simulink library "halout"  (R2021b)
settings: Solver=VariableStepAuto  StartTime=0.0  StopTime=10.0  RelTol=1e-3
undefined symbols (not defined in the file): C_TASK_5MS_S, FALSE, KHAL_CAN1FD1APS3E2E_flg, KHAL_CAN1FD1APS3TxReq_flg, KHAL_CAN1FD1VCU2E2E_flg, KHAL_CAN1FD1VCU2TxReq_flg, KHAL_CAN1FD1VCU3E2E_flg, KHAL_CAN1FD1VCU3TxReq_flg, KHAL_CAN1TxReq_flg, KHAL_CAN1VMCFCM1E2E_flg, KHAL_CAN1VMCFCM1TxReq_flg, KHAL_CAN2TxReq_flg, KHAL_CAN3FD3VCU1toNIDECTxReq_flg, KHAL_CAN3FD3VCU1TxReq_flg, KHAL_CAN3FD3VCU2E2E_flg, KHAL_CAN3FD3VCU2toNIDECE2E_flg, KHAL_CAN3FD3VCU2toNIDECTxReq_flg, KHAL_CAN3FD3VCU2TxReq_flg, KHAL_CAN3TxReq_flg, KHAL_CAN4FD4CE1000E2E_flg, KHAL_CAN4FD4CE1000TxReq_flg, KHAL_CAN4TxReq_flg, KHAL_CAN5TxReq_flg, KHAL_CAN6FD6APS3E2E_flg, KHAL_CAN6FD6APS3TxReq_flg, KHAL_CAN6FD6VCU2E2E_flg, KHAL_CAN6FD6VCU2TxReq_flg, KHAL_CAN6TxReq_flg, ONE_INT, TRUE, ZERO_INT
libraries: FVT_lib x551, simulink x244
(part 19 of 26)

== system halout/HAL_OUT/CAN3/FD3_BCM1_0x216/Dimmer ==
  Dimmer : Inport
  Data Type Conversion : DataTypeConversion  OutDataTypeStr=uint8  RndMeth=Round
  CAN3_Dimmer : Outport
  wires:
  Data Type Conversion/1 -> CAN3_Dimmer/1
  Dimmer/1 -> Data Type Conversion/1

== system halout/HAL_OUT/CAN3/FD3_BCM1_0x216/DimmerEN ==
  DimmerEN : Inport
  Data Type Conversion : DataTypeConversion  OutDataTypeStr=uint8  RndMeth=Round
  CAN3_DimmerEN : Outport
  wires:
  Data Type Conversion/1 -> CAN3_DimmerEN/1
  DimmerEN/1 -> Data Type Conversion/1

== system halout/HAL_OUT/CAN3/FD3_BCM1_0x216/DoorLockIND ==
  DoorLockIND : Inport
  Data Type Conversion : DataTypeConversion  OutDataTypeStr=uint8  RndMeth=Round
  CAN3_DoorLockIND : Outport
  wires:
  Data Type Conversion/1 -> CAN3_DoorLockIND/1
  DoorLockIND/1 -> Data Type Conversion/1

== system halout/HAL_OUT/CAN3/FD3_BCM1_0x216/DrDoorSW ==
  DrDoorSW : Inport
  Data Type Conversion : DataTypeConversion  OutDataTypeStr=uint8  RndMeth=Round
  CAN3_DrDoorSW : Outport
  wires:
  Data Type Conversion/1 -> CAN3_DrDoorSW/1
  DrDoorSW/1 -> Data Type Conversion/1

== system halout/HAL_OUT/CAN3/FD3_BCM1_0x216/FrChargingDoorCtrl ==
  FrChargingDoorCtrl : Inport
  Data Type Conversion : DataTypeConversion  OutDataTypeStr=uint8  RndMeth=Round
  CAN3_Fr_ChargingDoorCtrl : Outport
  wires:
  Data Type Conversion/1 -> CAN3_Fr_ChargingDoorCtrl/1
  FrChargingDoorCtrl/1 -> Data Type Conversion/1

== system halout/HAL_OUT/CAN3/FD3_BCM1_0x216/FrFogLamp ==
  FrFogLamp : Inport
  Data Type Conversion : DataTypeConversion  OutDataTypeStr=uint8  RndMeth=Round
  CAN3_Fr_FogLamp : Outport
  wires:
  Data Type Conversion/1 -> CAN3_Fr_FogLamp/1
  FrFogLamp/1 -> Data Type Conversion/1

== system halout/HAL_OUT/CAN3/FD3_BCM1_0x216/FrWiperH ==
  FrWiperH : Inport
  Data Type Conversion : DataTypeConversion  OutDataTypeStr=uint8  RndMeth=Round
  CAN3_Fr_Wiper_H : Outport
  wires:
  Data Type Conversion/1 -> CAN3_Fr_Wiper_H/1
  FrWiperH/1 -> Data Type Conversion/1

== system halout/HAL_OUT/CAN3/FD3_BCM1_0x216/FrWiperL ==
  FrWiperL : Inport
  Data Type Conversion : DataTypeConversion  OutDataTypeStr=uint8  RndMeth=Round
  CAN3_Fr_Wiper_L : Outport
  wires:
  Data Type Conversion/1 -> CAN3_Fr_Wiper_L/1
  FrWiperL/1 -> Data Type Conversion/1

== system halout/HAL_OUT/CAN3/FD3_BCM1_0x216/HBeam ==
  HBeam : Inport
  Data Type Conversion : DataTypeConversion  OutDataTypeStr=uint8  RndMeth=Round
  CAN3_H_Beam : Outport
  wires:
  Data Type Conversion/1 -> CAN3_H_Beam/1
  HBeam/1 -> Data Type Conversion/1

== system halout/HAL_OUT/CAN3/FD3_BCM1_0x216/HazardSW ==
  HazardSW : Inport
  Data Type Conversion : DataTypeConversion  OutDataTypeStr=uint8  RndMeth=Round
  CAN3_HazardSW : Outport
  wires:
  Data Type Conversion/1 -> CAN3_HazardSW/1
  HazardSW/1 -> Data Type Conversion/1

== system halout/HAL_OUT/CAN3/FD3_BCM1_0x216/HoodSW ==
  HoodSW : Inport
  Data Type Conversion : DataTypeConversion  OutDataTypeStr=uint8  RndMeth=Round
  CAN3_HoodSW : Outport
  wires:
  Data Type Conversion/1 -> CAN3_HoodSW/1
  HoodSW/1 -> Data Type Conversion/1

== system halout/HAL_OUT/CAN3/FD3_BCM1_0x216/HornCtrl ==
  HornCtrl : Inport
  Data Type Conversion : DataTypeConversion  OutDataTypeStr=uint8  RndMeth=Round
  CAN3_HornCtrl : Outport
  wires:
  Data Type Conversion/1 -> CAN3_HornCtrl/1
  HornCtrl/1 -> Data Type Conversion/1

== system halout/HAL_OUT/CAN3/FD3_BCM1_0x216/LAPMWdwEnable ==
  LAPMWdwEnable : Inport
  Data Type Conversion : DataTypeConversion  OutDataTypeStr=uint8  RndMeth=Round
  CAN3_L_APM_WdwEnable : Outport
  wires:
  Data Type Conversion/1 -> CAN3_L_APM_WdwEnable/1
  LAPMWdwEnable/1 -> Data Type Conversion/1

== system halout/HAL_OUT/CAN3/FD3_BCM1_0x216/LBSD ==
  LBSD : Inport
  Data Type Conversion : DataTypeConversion  OutDataTypeStr=uint8  RndMeth=Round
  CAN3_LBSD : Outport
  wires:
  Data Type Conversion/1 -> CAN3_LBSD/1
  LBSD/1 -> Data Type Conversion/1

== system halout/HAL_OUT/CAN3/FD3_BCM1_0x216/LBeam ==
  LBeam : Inport
  Data Type Conversion : DataTypeConversion  OutDataTypeStr=uint8  RndMeth=Round
  CAN3_L_Beam : Outport
  wires:
  Data Type Conversion/1 -> CAN3_L_Beam/1
  LBeam/1 -> Data Type Conversion/1

== system halout/HAL_OUT/CAN3/FD3_BCM1_0x216/LDRL ==
  LDRL : Inport
  Data Type Conversion : DataTypeConversion  OutDataTypeStr=uint8  RndMeth=Round
  CAN3_LDRL : Outport
  wires:
  Data Type Conversion/1 -> CAN3_LDRL/1
  LDRL/1 -> Data Type Conversion/1

== system halout/HAL_OUT/CAN3/FD3_BCM1_0x216/LTurnLP ==
  LTurnLP : Inport
  Data Type Conversion : DataTypeConversion  OutDataTypeStr=uint8  RndMeth=Round
  CAN3_LTurnLP : Outport
  wires:
  Data Type Conversion/1 -> CAN3_LTurnLP/1
  LTurnLP/1 -> Data Type Conversion/1

== system halout/HAL_OUT/CAN3/FD3_BCM1_0x216/LockSetting ==
  LockSetting : Inport
  Data Type Conversion : DataTypeConversion  OutDataTypeStr=uint8  RndMeth=Round
  CAN3_LockSetting : Outport
  wires:
  Data Type Conversion/1 -> CAN3_LockSetting/1
  LockSetting/1 -> Data Type Conversion/1

== system halout/HAL_OUT/CAN3/FD3_BCM1_0x216/MirrorCtrl ==
  MirrorCtrl : Inport
  Data Type Conversion : DataTypeConversion  OutDataTypeStr=uint8  RndMeth=Round
  CAN3_MirrorCtrl : Outport
  wires:
  Data Type Conversion/1 -> CAN3_MirrorCtrl/1
  MirrorCtrl/1 -> Data Type Conversion/1

== system halout/HAL_OUT/CAN3/FD3_BCM1_0x216/MirrorDefog ==
  MirrorDefog : Inport
  Data Type Conversion : DataTypeConversion  OutDataTypeStr=uint8  RndMeth=Round
  CAN3_MirrorDefog : Outport
  wires:
  Data Type Conversion/1 -> CAN3_MirrorDefog/1
  MirrorDefog/1 -> Data Type Conversion/1

== system halout/HAL_OUT/CAN3/FD3_BCM1_0x216/PosLamp ==
  PosLamp : Inport
  Data Type Conversion : DataTypeConversion  OutDataTypeStr=uint8  RndMeth=Round
  CAN3_PosLamp : Outport
  wires:
  Data Type Conversion/1 -> CAN3_PosLamp/1
  PosLamp/1 -> Data Type Conversion/1

== system halout/HAL_OUT/CAN3/FD3_BCM1_0x216/PsDoorSW ==
  PsDoorSW : Inport
  Data Type Conversion : DataTypeConversion  OutDataTypeStr=uint8  RndMeth=Round
  CAN3_PsDoorSW : Outport
  wires:
  Data Type Conversion/1 -> CAN3_PsDoorSW/1
  PsDoorSW/1 -> Data Type Conversion/1

== system halout/HAL_OUT/CAN3/FD3_BCM1_0x216/RBSD ==
  RBSD : Inport
  Data Type Conversion : DataTypeConversion  OutDataTypeStr=uint8  RndMeth=Round
  CAN3_RBSD : Outport
  wires:
  Data Type Conversion/1 -> CAN3_RBSD/1
  RBSD/1 -> Data Type Conversion/1

== system halout/HAL_OUT/CAN3/FD3_BCM1_0x216/RDRL ==
  RDRL : Inport
  Data Type Conversion : DataTypeConversion  OutDataTypeStr=uint8  RndMeth=Round
  CAN3_RDRL : Outport
  wires:
  Data Type Conversion/1 -> CAN3_RDRL/1
  RDRL/1 -> Data Type Conversion/1

== system halout/HAL_OUT/CAN3/FD3_BCM1_0x216/RLDoorSW ==
  RLDoorSW : Inport
  Data Type Conversion : DataTypeConversion  OutDataTypeStr=uint8  RndMeth=Round
  CAN3_RLDoorSW : Outport
  wires:
  Data Type Conversion/1 -> CAN3_RLDoorSW/1
  RLDoorSW/1 -> Data Type Conversion/1

== system halout/HAL_OUT/CAN3/FD3_BCM1_0x216/RRDoorSW ==
  RRDoorSW : Inport
  Data Type Conversion : DataTypeConversion  OutDataTypeStr=uint8  RndMeth=Round
  CAN3_RRDoorSW : Outport
  wires:
  Data Type Conversion/1 -> CAN3_RRDoorSW/1
  RRDoorSW/1 -> Data Type Conversion/1

== system halout/HAL_OUT/CAN3/FD3_BCM1_0x216/RTurnLP ==
  RTurnLP : Inport
  Data Type Conversion : DataTypeConversion  OutDataTypeStr=uint8  RndMeth=Round
  CAN3_RTurnLP : Outport
  wires:
  Data Type Conversion/1 -> CAN3_RTurnLP/1
  RTurnLP/1 -> Data Type Conversion/1

== system halout/HAL_OUT/CAN3/FD3_BCM1_0x216/ReverseLamp ==
  ReverseLamp : Inport
  Data Type Conversion : DataTypeConversion  OutDataTypeStr=uint8  RndMeth=Round
  CAN3_ReverseLamp : Outport
  wires:
  Data Type Conversion/1 -> CAN3_ReverseLamp/1
  ReverseLamp/1 -> Data Type Conversion/1

== system halout/HAL_OUT/CAN3/FD3_BCM1_0x216/RoomLampH ==
  RoomLampH : Inport
  Data Type Conversion : DataTypeConversion  OutDataTypeStr=uint8  RndMeth=Round
  CAN3_RoomLampH : Outport
  wires:
  Data Type Conversion/1 -> CAN3_RoomLampH/1
  RoomLampH/1 -> Data Type Conversion/1

== system halout/HAL_OUT/CAN3/FD3_BCM1_0x216/RoomLampL ==
  RoomLampL : Inport
  Data Type Conversion : DataTypeConversion  OutDataTypeStr=uint8  RndMeth=Round
  CAN3_RoomLampL : Outport
  wires:
  Data Type Conversion/1 -> CAN3_RoomLampL/1
  RoomLampL/1 -> Data Type Conversion/1

== system halout/HAL_OUT/CAN3/FD3_BCM1_0x216/RrChargingDoorCtrl ==
  RrChargingDoorCtrl : Inport
  Data Type Conversion : DataTypeConversion  OutDataTypeStr=uint8  RndMeth=Round
  CAN3_Rr_ChargingDoorCtrl : Outport
  wires:
  Data Type Conversion/1 -> CAN3_Rr_ChargingDoorCtrl/1
  RrChargingDoorCtrl/1 -> Data Type Conversion/1

== system halout/HAL_OUT/CAN3/FD3_BCM1_0x216/RrDefog ==
  RrDefog : Inport
  Data Type Conversion : DataTypeConversion  OutDataTypeStr=uint8  RndMeth=Round
  CAN3_Rr_Defog : Outport
  wires:
  Data Type Conversion/1 -> CAN3_Rr_Defog/1
  RrDefog/1 -> Data Type Conversion/1

== system halout/HAL_OUT/CAN3/FD3_BCM1_0x216/RrFogLamp ==
  RrFogLamp : Inport
  Data Type Conversion : DataTypeConversion  OutDataTypeStr=uint8  RndMeth=Round
  CAN3_Rr_FogLamp : Outport
  wires:
  Data Type Conversion/1 -> CAN3_Rr_FogLamp/1
  RrFogLamp/1 -> Data Type Conversion/1

== system halout/HAL_OUT/CAN3/FD3_BCM1_0x216/RrWiper ==
  RrWiper : Inport
  Data Type Conversion : DataTypeConversion  OutDataTypeStr=uint8  RndMeth=Round
  CAN3_Rr_Wiper : Outport
  wires:
  Data Type Conversion/1 -> CAN3_Rr_Wiper/1
  RrWiper/1 -> Data Type Conversion/1

== system halout/HAL_OUT/CAN3/FD3_BCM1_0x216/TailgateHDSW ==
  TailgateHDSW : Inport
  Data Type Conversion : DataTypeConversion  OutDataTypeStr=uint8  RndMeth=Round
  CAN3_TailgateHDSW : Outport
  wires:
  Data Type Conversion/1 -> CAN3_TailgateHDSW/1
  TailgateHDSW/1 -> Data Type Conversion/1

== system halout/HAL_OUT/CAN3/FD3_BCM1_0x216/TailgateRemote ==
  TailgateRemote : Inport
  Data Type Conversion : DataTypeConversion  OutDataTypeStr=uint8  RndMeth=Round
  CAN3_TailgateRemote : Outport
  wires:
  Data Type Conversion/1 -> CAN3_TailgateRemote/1
  TailgateRemote/1 -> Data Type Conversion/1

== system halout/HAL_OUT/CAN3/FD3_BCM1_0x216/TailgateSW ==
  TailgateSW : Inport
  Data Type Conversion : DataTypeConversion  OutDataTypeStr=uint8  RndMeth=Round
  CAN3_Tailgate_SW : Outport
  wires:
  Data Type Conversion/1 -> CAN3_Tailgate_SW/1
  TailgateSW/1 -> Data Type Conversion/1

== system halout/HAL_OUT/CAN3/FD3_BCM1_0x216/TrunkRel ==
  TrunkRel : Inport
  Data Type Conversion : DataTypeConversion  OutDataTypeStr=uint8  RndMeth=Round
  CAN3_TrunkRel : Outport
  wires:
  Data Type Conversion/1 -> CAN3_TrunkRel/1
  TrunkRel/1 -> Data Type Conversion/1

== system halout/HAL_OUT/CAN3/FD3_BCM1_0x216/WasherCtrl ==
  WasherCtrl : Inport
  Data Type Conversion : DataTypeConversion  OutDataTypeStr=uint8  RndMeth=Round
  CAN3_WasherCtrl : Outport
  wires:
  Data Type Conversion/1 -> CAN3_WasherCtrl/1
  WasherCtrl/1 -> Data Type Conversion/1

== system halout/HAL_OUT/CAN3/FD3_BCM1_0x216/WiperFixMode ==
  WiperFixMode : Inport
  Data Type Conversion : DataTypeConversion  OutDataTypeStr=uint8  RndMeth=Round
  CAN3_WiperFixMode : Outport
  wires:
  Data Type Conversion/1 -> CAN3_WiperFixMode/1
  WiperFixMode/1 -> Data Type Conversion/1

== system halout/HAL_OUT/CAN3/FD3_C100_0_0x182/BatteryMode ==
  BatteryMode : Inport
  Data Type Conversion : DataTypeConversion  OutDataTypeStr=uint8  RndMeth=Round
  CAN3_BatteryMode : Outport
  wires:
  Data Type Conversion/1 -> CAN3_BatteryMode/1
  BatteryMode/1 -> Data Type Conversion/1

== system halout/HAL_OUT/CAN3/FD3_C100_0_0x182/FrCoolantflow ==
  FrCoolantflow : Inport
  Data Type Conversion : DataTypeConversion  OutDataTypeStr=uint8  RndMeth=Round
  convert_out : FVT_lib/hal/convert_out  gain=0.25  offset=0
  CAN3_Fr_Coolantflow : Outport
  wires:
  Data Type Conversion/1 -> CAN3_Fr_Coolantflow/1
  convert_out/1 -> Data Type Conversion/1
  FrCoolantflow/1 -> convert_out/1

== system halout/HAL_OUT/CAN3/FD3_C100_0_0x182/FrCoolanttemp ==
  FrCoolanttemp : Inport
  Data Type Conversion : DataTypeConversion  OutDataTypeStr=uint16  RndMeth=Round
  convert_out : FVT_lib/hal/convert_out  gain=1  offset=-40
  CAN3_Fr_Coolanttemp : Outport
  wires:
  Data Type Conversion/1 -> CAN3_Fr_Coolanttemp/1
  convert_out/1 -> Data Type Conversion/1
  FrCoolanttemp/1 -> convert_out/1

== system halout/HAL_OUT/CAN3/FD3_C100_0_0x182/RrCoolantflow ==
  RrCoolantflow : Inport
  Data Type Conversion : DataTypeConversion  OutDataTypeStr=uint8  RndMeth=Round
  convert_out : FVT_lib/hal/convert_out  gain=0.25  offset=0
  CAN3_Rr_Coolantflow : Outport
  wires:
  Data Type Conversion/1 -> CAN3_Rr_Coolantflow/1
  convert_out/1 -> Data Type Conversion/1
  RrCoolantflow/1 -> convert_out/1

== system halout/HAL_OUT/CAN3/FD3_C100_0_0x182/RrCoolanttemp ==
  RrCoolanttemp : Inport
  Data Type Conversion : DataTypeConversion  OutDataTypeStr=uint16  RndMeth=Round
  convert_out : FVT_lib/hal/convert_out  gain=1  offset=-40
  CAN3_Rr_Coolanttemp : Outport
  wires:
  Data Type Conversion/1 -> CAN3_Rr_Coolanttemp/1
  convert_out/1 -> Data Type Conversion/1
  RrCoolanttemp/1 -> convert_out/1

== system halout/HAL_OUT/CAN3/FD3_C100_0_0x182/sigCbnPTCPwrAct ==
  sigCbnPTCPwrAct : Inport
  Data Type Conversion : DataTypeConversion  OutDataTypeStr=uint8  RndMeth=Round
  convert_out : FVT_lib/hal/convert_out  gain=50  offset=0
  CAN3_sigCbnPTCPwrAct : Outport
  wires:
  Data Type Conversion/1 -> CAN3_sigCbnPTCPwrAct/1
  convert_out/1 -> Data Type Conversion/1
  sigCbnPTCPwrAct/1 -> convert_out/1

== system halout/HAL_OUT/CAN3/FD3_V2L1_0x374/FDCV2LOBCExtrV2LCmd ==
  FDCV2LOBCExtrV2LCmd : Inport
  Data Type Conversion : DataTypeConversion  OutDataTypeStr=uint8  RndMeth=Round
  CAN3_FDC_V2L_OBCExtrV2L_Cmd : Outport
  wires:
  Data Type Conversion/1 -> CAN3_FDC_V2L_OBCExtrV2L_Cmd/1
  FDCV2LOBCExtrV2LCmd/1 -> Data Type Conversion/1

== system halout/HAL_OUT/CAN3/FD3_V2L1_0x374/FDCV2LOBCIntrV2LCmd ==
  FDCV2LOBCIntrV2LCmd : Inport
  Data Type Conversion : DataTypeConversion  OutDataTypeStr=uint8  RndMeth=Round
  CAN3_FDC_V2L_OBCIntrV2L_Cmd : Outport
  wires:
  Data Type Conversion/1 -> CAN3_FDC_V2L_OBCIntrV2L_Cmd/1
  FDCV2LOBCIntrV2LCmd/1 -> Data Type Conversion/1

== system halout/HAL_OUT/CAN3/FD3_V2L1_0x374/ReqOBCV2LEna ==
  ReqOBCV2LEna : Inport
  Data Type Conversion : DataTypeConversion  OutDataTypeStr=uint8  RndMeth=Round
  CAN3_Req_OBCV2LEna : Outport
  wires:
  Data Type Conversion/1 -> CAN3_Req_OBCV2LEna/1
  ReqOBCV2LEna/1 -> Data Type Conversion/1

== system halout/HAL_OUT/CAN3/FD3_V2L1_0x374/ReqV2LIVIPopup ==
  ReqV2LIVIPopup : Inport
  Data Type Conversion : DataTypeConversion  OutDataTypeStr=uint8  RndMeth=Round
  CAN3_Req_V2L_IVI_Popup : Outport
  wires:
  Data Type Conversion/1 -> CAN3_Req_V2L_IVI_Popup/1
  ReqV2LIVIPopup/1 -> Data Type Conversion/1

== system halout/HAL_OUT/CAN3/FD3_V2L1_0x374/ReqV2LSwOn ==
  ReqV2LSwOn : Inport
  Data Type Conversion : DataTypeConversion  OutDataTypeStr=uint8  RndMeth=Round
  CAN3_Req_V2LSwOn : Outport
  wires:
  Data Type Conversion/1 -> CAN3_Req_V2LSwOn/1
  ReqV2LSwOn/1 -> Data Type Conversion/1

== system halout/HAL_OUT/CAN3/FD3_VCU0_0x1F0/EVCCAplusPwrUpReq ==
  EVCCAplusPwrUpReq : Inport
  Data Type Conversion : DataTypeConversion  OutDataTypeStr=uint8  RndMeth=Round
  CAN3_EVCCAplusPwrUpReq : Outport
  wires:
  Data Type Conversion/1 -> CAN3_EVCCAplusPwrUpReq/1
  EVCCAplusPwrUpReq/1 -> Data Type Conversion/1

== system halout/HAL_OUT/CAN3/FD3_VCU0_0x1F0/FDADC12VDet ==
  FDADC12VDet : Inport
  Data Type Conversion : DataTypeConversion  OutDataTypeStr=uint8  RndMeth=Round
  convert_out : FVT_lib/hal/convert_out  gain=0.1  offset=0
  CAN3_FDADC12VDet : Outport
  wires:
  Data Type Conversion/1 -> CAN3_FDADC12VDet/1
  convert_out/1 -> Data Type Conversion/1
  FDADC12VDet/1 -> convert_out/1

== system halout/HAL_OUT/CAN3/FD3_VCU0_0x1F0/FDADC12VDetAvg ==
  FDADC12VDetAvg : Inport
  Data Type Conversion : DataTypeConversion  OutDataTypeStr=uint8  RndMeth=Round
  convert_out : FVT_lib/hal/convert_out  gain=0.1  offset=0
  CAN3_FDADC12VDetAvg : Outport
  wires:
  Data Type Conversion/1 -> CAN3_FDADC12VDetAvg/1
  convert_out/1 -> Data Type Conversion/1
  FDADC12VDetAvg/1 -> convert_out/1

== system halout/HAL_OUT/CAN3/FD3_VCU0_0x1F0/FDCSYSPmicBootPath ==
  FDCSYSPmicBootPath : Inport
  Data Type Conversion : DataTypeConversion  OutDataTypeStr=uint32  RndMeth=Round
  CAN3_FDC_SYS_PmicBootPath : Outport
  wires:
  Data Type Conversion/1 -> CAN3_FDC_SYS_PmicBootPath/1
  FDCSYSPmicBootPath/1 -> Data Type Conversion/1

== system halout/HAL_OUT/CAN3/FD3_VCU0_0x1F0/FDCVCUActMaxSlideRateSta ==
  FDCVCUActMaxSlideRateSta : Inport
  Data Type Conversion : DataTypeConversion  OutDataTypeStr=uint16  RndMeth=Round
  convert_out : FVT_lib/hal/convert_out  gain=0.01  offset=-150
  CAN3_FDC_VCU_ActMaxSlideRate_Sta : Outport
  wires:
  Data Type Conversion/1 -> CAN3_FDC_VCU_ActMaxSlideRate_Sta/1
  convert_out/1 -> Data Type Conversion/1
  FDCVCUActMaxSlideRateSta/1 -> convert_out/1

== system halout/HAL_OUT/CAN3/FD3_VCU0_0x1F0/FDCVCUAllowMovThdOTASta ==
  FDCVCUAllowMovThdOTASta : Inport
  Data Type Conversion : DataTypeConversion  OutDataTypeStr=uint8  RndMeth=Round
  CAN3_FDC_VCU_AllowMovThd_OTA_Sta : Outport
  wires:
  Data Type Conversion/1 -> CAN3_FDC_VCU_AllowMovThd_OTA_Sta/1
  FDCVCUAllowMovThdOTASta/1 -> Data Type Conversion/1

== system halout/HAL_OUT/CAN3/FD3_VCU0_0x1F0/FDCVCUBOSEnableSta ==
  FDCVCUBOSEnableSta : Inport
  Data Type Conversion : DataTypeConversion  OutDataTypeStr=uint8  RndMeth=Round
  CAN3_FDC_VCU_BOSEnable_Sta : Outport
  wires:
  Data Type Conversion/1 -> CAN3_FDC_VCU_BOSEnable_Sta/1
  FDCVCUBOSEnableSta/1 -> Data Type Conversion/1

== system halout/HAL_OUT/CAN3/FD3_VCU0_0x1F0/FDCVCUBrakeSigMatrixSta ==
  FDCVCUBrakeSigMatrixSta : Inport
  Data Type Conversion : DataTypeConversion  OutDataTypeStr=uint8  RndMeth=Round
  CAN3_FDC_VCU_BrakeSigMatrix_Sta : Outport
  wires:
  Data Type Conversion/1 -> CAN3_FDC_VCU_BrakeSigMatrix_Sta/1
  FDCVCUBrakeSigMatrixSta/1 -> Data Type Conversion/1

== system halout/HAL_OUT/CAN3/FD3_VCU0_0x1F0/FDCVCUBrkPedalPosStaSta ==
  FDCVCUBrkPedalPosStaSta : Inport
  Data Type Conversion : DataTypeConversion  OutDataTypeStr=uint8  RndMeth=Round
  CAN3_FDC_VCU_BrkPedalPosSta_Sta : Outport
  wires:
  Data Type Conversion/1 -> CAN3_FDC_VCU_BrkPedalPosSta_Sta/1
  FDCVCUBrkPedalPosStaSta/1 -> Data Type Conversion/1

== system halout/HAL_OUT/CAN3/FD3_VCU0_0x1F0/FDCVCUCANBrkSW2StaSta ==
  FDCVCUCANBrkSW2StaSta : Inport
  Data Type Conversion : DataTypeConversion  OutDataTypeStr=uint8  RndMeth=Round
  CAN3_FDC_VCU_CANBrkSW2Sta_Sta : Outport
  wires:
  Data Type Conversion/1 -> CAN3_FDC_VCU_CANBrkSW2Sta_Sta/1
  FDCVCUCANBrkSW2StaSta/1 -> Data Type Conversion/1

== system halout/HAL_OUT/CAN3/FD3_VCU0_0x1F0/FDCVCUDTCCarouselSta ==
  FDCVCUDTCCarouselSta : Inport
  Data Type Conversion : DataTypeConversion  OutDataTypeStr=uint8  RndMeth=Round
  CAN3_FDC_VCU_DTCCarousel_Sta : Outport
  wires:
  Data Type Conversion/1 -> CAN3_FDC_VCU_DTCCarousel_Sta/1
  FDCVCUDTCCarouselSta/1 -> Data Type Conversion/1

== system halout/HAL_OUT/CAN3/FD3_VCU0_0x1F0/FDCVCUEAPS1MinSta ==
  FDCVCUEAPS1MinSta : Inport
  Data Type Conversion : DataTypeConversion  OutDataTypeStr=uint8  RndMeth=Round
  convert_out : FVT_lib/hal/convert_out  gain=0.4  offset=0
  CAN3_FDC_VCU_EAPS1Min_Sta : Outport
  wires:
  Data Type Conversion/1 -> CAN3_FDC_VCU_EAPS1Min_Sta/1
  convert_out/1 -> Data Type Conversion/1
  FDCVCUEAPS1MinSta/1 -> convert_out/1

== system halout/HAL_OUT/CAN3/FD3_VCU0_0x1F0/FDCVCUEAPS1RawSta ==
  FDCVCUEAPS1RawSta : Inport
  Data Type Conversion : DataTypeConversion  OutDataTypeStr=uint8  RndMeth=Round
  convert_out : FVT_lib/hal/convert_out  gain=0.4  offset=0
  CAN3_FDC_VCU_EAPS1Raw_Sta : Outport
  wires:
  Data Type Conversion/1 -> CAN3_FDC_VCU_EAPS1Raw_Sta/1
  convert_out/1 -> Data Type Conversion/1
  FDCVCUEAPS1RawSta/1 -> convert_out/1

== system halout/HAL_OUT/CAN3/FD3_VCU0_0x1F0/FDCVCUEAPS2MinSta ==
  FDCVCUEAPS2MinSta : Inport
  Data Type Conversion : DataTypeConversion  OutDataTypeStr=uint8  RndMeth=Round
  convert_out : FVT_lib/hal/convert_out  gain=0.4  offset=0
  CAN3_FDC_VCU_EAPS2Min_Sta : Outport
  wires:
  Data Type Conversion/1 -> CAN3_FDC_VCU_EAPS2Min_Sta/1
  convert_out/1 -> Data Type Conversion/1
  FDCVCUEAPS2MinSta/1 -> convert_out/1

== system halout/HAL_OUT/CAN3/FD3_VCU0_0x1F0/FDCVCUEAPS2RawSta ==
  FDCVCUEAPS2RawSta : Inport
  Data Type Conversion : DataTypeConversion  OutDataTypeStr=uint8  RndMeth=Round
  convert_out : FVT_lib/hal/convert_out  gain=0.4  offset=0
  CAN3_FDC_VCU_EAPS2Raw_Sta : Outport
  wires:
  Data Type Conversion/1 -> CAN3_FDC_VCU_EAPS2Raw_Sta/1
  convert_out/1 -> Data Type Conversion/1
  FDCVCUEAPS2RawSta/1 -> convert_out/1

== system halout/HAL_OUT/CAN3/FD3_VCU0_0x1F0/FDCVCUForcePCmd ==
  FDCVCUForcePCmd : Inport
  Data Type Conversion : DataTypeConversion  OutDataTypeStr=uint8  RndMeth=Round
  CAN3_FDC_VCU_ForceP_Cmd : Outport
  wires:
  Data Type Conversion/1 -> CAN3_FDC_VCU_ForceP_Cmd/1
  FDCVCUForcePCmd/1 -> Data Type Conversion/1

== system halout/HAL_OUT/CAN3/FD3_VCU0_0x1F0/FDCVCUFrFirstOrderInpTs ==
  FDCVCUFrFirstOrderInpTs : Inport
  Data Type Conversion : DataTypeConversion  OutDataTypeStr=uint8  RndMeth=Round
  convert_out : FVT_lib/hal/convert_out  gain=0.01  offset=0
  CAN3_FDC_VCU_FrFirstOrderInpTs : Outport
  wires:
  Data Type Conversion/1 -> CAN3_FDC_VCU_FrFirstOrderInpTs/1
  convert_out/1 -> Data Type Conversion/1
  FDCVCUFrFirstOrderInpTs/1 -> convert_out/1

== system halout/HAL_OUT/CAN3/FD3_VCU0_0x1F0/FDCVCUFrRateLimitDecSta ==
  FDCVCUFrRateLimitDecSta : Inport
  Data Type Conversion : DataTypeConversion  OutDataTypeStr=uint16  RndMeth=Round
  convert_out : FVT_lib/hal/convert_out  gain=2  offset=-131070
  CAN3_FDC_VCU_FrRateLimitDec_Sta : Outport
  wires:
  Data Type Conversion/1 -> CAN3_FDC_VCU_FrRateLimitDec_Sta/1
  convert_out/1 -> Data Type Conversion/1
  FDCVCUFrRateLimitDecSta/1 -> convert_out/1

== system halout/HAL_OUT/CAN3/FD3_VCU0_0x1F0/FDCVCUFrRateLimitIncSta ==
  FDCVCUFrRateLimitIncSta : Inport
  Data Type Conversion : DataTypeConversion  OutDataTypeStr=uint16  RndMeth=Round
  convert_out : FVT_lib/hal/convert_out  gain=2  offset=0
  CAN3_FDC_VCU_FrRateLimitInc_Sta : Outport
  wires:
  Data Type Conversion/1 -> CAN3_FDC_VCU_FrRateLimitInc_Sta/1
  convert_out/1 -> Data Type Conversion/1
  FDCVCUFrRateLimitIncSta/1 -> convert_out/1

== system halout/HAL_OUT/CAN3/FD3_VCU0_0x1F0/FDCVCULVChrgFreqCntSta ==
  FDCVCULVChrgFreqCntSta : Inport
  Data Type Conversion : DataTypeConversion  OutDataTypeStr=uint8  RndMeth=Round
  CAN3_FDC_VCU_LVChrgFreqCnt_Sta : Outport
  wires:
  Data Type Conversion/1 -> CAN3_FDC_VCU_LVChrgFreqCnt_Sta/1
  FDCVCULVChrgFreqCntSta/1 -> Data Type Conversion/1

== system halout/HAL_OUT/CAN3/FD3_VCU0_0x1F0/FDCVCULVStaDropQukCntSta ==
  FDCVCULVStaDropQukCntSta : Inport
  Data Type Conversion : DataTypeConversion  OutDataTypeStr=uint8  RndMeth=Round
  CAN3_FDC_VCU_LVStaDropQukCnt_Sta : Outport
  wires:
  Data Type Conversion/1 -> CAN3_FDC_VCU_LVStaDropQukCnt_Sta/1
  FDCVCULVStaDropQukCntSta/1 -> Data Type Conversion/1

== system halout/HAL_OUT/CAN3/FD3_VCU0_0x1F0/FDCVCULowIdleAccPedalSta ==
  FDCVCULowIdleAccPedalSta : Inport
  Data Type Conversion : DataTypeConversion  OutDataTypeStr=uint8  RndMeth=Round
  CAN3_FDC_VCU_LowIdleAccPedal_Sta : Outport
  wires:
  Data Type Conversion/1 -> CAN3_FDC_VCU_LowIdleAccPedal_Sta/1
  FDCVCULowIdleAccPedalSta/1 -> Data Type Conversion/1

== system halout/HAL_OUT/CAN3/FD3_VCU0_0x1F0/FDCVCUOTAPwrReqOFFChkSta ==
  FDCVCUOTAPwrReqOFFChkSta : Inport
  Data Type Conversion : DataTypeConversion  OutDataTypeStr=uint8  RndMeth=Round
  CAN3_FDC_VCU_OTAPwrReqOFFChk_Sta : Outport
  wires:
  Data Type Conversion/1 -> CAN3_FDC_VCU_OTAPwrReqOFFChk_Sta/1
  FDCVCUOTAPwrReqOFFChkSta/1 -> Data Type Conversion/1

== system halout/HAL_OUT/CAN3/FD3_VCU0_0x1F0/FDCVCUOTAPwrReqStdChkSta ==
  FDCVCUOTAPwrReqStdChkSta : Inport
  Data Type Conversion : DataTypeConversion  OutDataTypeStr=uint8  RndMeth=Round
  CAN3_FDC_VCU_OTAPwrReqStdChk_Sta : Outport
  wires:
  Data Type Conversion/1 -> CAN3_FDC_VCU_OTAPwrReqStdChk_Sta/1
  FDCVCUOTAPwrReqStdChkSta/1 -> Data Type Conversion/1

== system halout/HAL_OUT/CAN3/FD3_VCU0_0x1F0/FDCVCUPwrReqOTASta ==
  FDCVCUPwrReqOTASta : Inport
  Data Type Conversion : DataTypeConversion  OutDataTypeStr=uint8  RndMeth=Round
  CAN3_FDC_VCU_PwrReq_OTA_Sta : Outport
  wires:
  Data Type Conversion/1 -> CAN3_FDC_VCU_PwrReq_OTA_Sta/1
  FDCVCUPwrReqOTASta/1 -> Data Type Conversion/1

== system halout/HAL_OUT/CAN3/FD3_VCU0_0x1F0/FDCVCURWDRDCActiveSta ==
  FDCVCURWDRDCActiveSta : Inport
  Data Type Conversion : DataTypeConversion  OutDataTypeStr=uint8  RndMeth=Round
  CAN3_FDC_VCU_RWDRDCActive_Sta : Outport
  wires:
  Data Type Conversion/1 -> CAN3_FDC_VCU_RWDRDCActive_Sta/1
  FDCVCURWDRDCActiveSta/1 -> Data Type Conversion/1

== system halout/HAL_OUT/CAN3/FD3_VCU0_0x1F0/FDCVCURegenTqLimitEnSta ==
  FDCVCURegenTqLimitEnSta : Inport
  Data Type Conversion : DataTypeConversion  OutDataTypeStr=uint8  RndMeth=Round
  CAN3_FDC_VCU_RegenTqLimitEn_Sta : Outport
  wires:
  Data Type Conversion/1 -> CAN3_FDC_VCU_RegenTqLimitEn_Sta/1
  FDCVCURegenTqLimitEnSta/1 -> Data Type Conversion/1

== system halout/HAL_OUT/CAN3/FD3_VCU0_0x1F0/FDCVCURrFirstOrderInpTs ==
  FDCVCURrFirstOrderInpTs : Inport
  Data Type Conversion : DataTypeConversion  OutDataTypeStr=uint8  RndMeth=Round
  convert_out : FVT_lib/hal/convert_out  gain=0.01  offset=0
  CAN3_FDC_VCU_RrFirstOrderInpTs : Outport
  wires:
  Data Type Conversion/1 -> CAN3_FDC_VCU_RrFirstOrderInpTs/1
  convert_out/1 -> Data Type Conversion/1
  FDCVCURrFirstOrderInpTs/1 -> convert_out/1

== system halout/HAL_OUT/CAN3/FD3_VCU0_0x1F0/FDCVCURrRateLimitDecSta ==
  FDCVCURrRateLimitDecSta : Inport
  Data Type Conversion : DataTypeConversion  OutDataTypeStr=uint16  RndMeth=Round
  convert_out : FVT_lib/hal/convert_out  gain=2  offset=-131070
  CAN3_FDC_VCU_RrRateLimitDec_Sta : Outport
  wires:
  Data Type Conversion/1 -> CAN3_FDC_VCU_RrRateLimitDec_Sta/1
  convert_out/1 -> Data Type Conversion/1
  FDCVCURrRateLimitDecSta/1 -> convert_out/1

== system halout/HAL_OUT/CAN3/FD3_VCU0_0x1F0/FDCVCURrRateLimitIncSta ==
  FDCVCURrRateLimitIncSta : Inport
  Data Type Conversion : DataTypeConversion  OutDataTypeStr=uint16  RndMeth=Round
  convert_out : FVT_lib/hal/convert_out  gain=2  offset=0
  CAN3_FDC_VCU_RrRateLimitInc_Sta : Outport
  wires:
  Data Type Conversion/1 -> CAN3_FDC_VCU_RrRateLimitInc_Sta/1
  convert_out/1 -> Data Type Conversion/1
  FDCVCURrRateLimitIncSta/1 -> convert_out/1

== system halout/HAL_OUT/CAN3/FD3_VCU0_0x1F0/FDCVCUSlideRegenLimTqSta ==
  FDCVCUSlideRegenLimTqSta : Inport
  Data Type Conversion : DataTypeConversion  OutDataTypeStr=uint16  RndMeth=Round
  convert_out : FVT_lib/hal/convert_out  gain=0.5  offset=-5300
  CAN3_FDC_VCU_SlideRegenLimTq_Sta : Outport
  wires:
  Data Type Conversion/1 -> CAN3_FDC_VCU_SlideRegenLimTq_Sta/1
  convert_out/1 -> Data Type Conversion/1
  FDCVCUSlideRegenLimTqSta/1 -> convert_out/1

== system halout/HAL_OUT/CAN3/FD3_VCU0_0x1F0/FDCVCUVehActSpdSta ==
  FDCVCUVehActSpdSta : Inport
  Data Type Conversion : DataTypeConversion  OutDataTypeStr=uint16  RndMeth=Round
  convert_out : FVT_lib/hal/convert_out  gain=0.01  offset=-300
  CAN3_FDC_VCU_VehActSpd_Sta : Outport
  wires:
  Data Type Conversion/1 -> CAN3_FDC_VCU_VehActSpd_Sta/1
  convert_out/1 -> Data Type Conversion/1
  FDCVCUVehActSpdSta/1 -> convert_out/1

== system halout/HAL_OUT/CAN3/FD3_VCU0_0x1F0/FDCVCUVehMalfunLevelSta ==
  FDCVCUVehMalfunLevelSta : Inport
  Data Type Conversion : DataTypeConversion  OutDataTypeStr=uint8  RndMeth=Round
  CAN3_FDC_VCU_VehMalfunLevel_Sta : Outport
  wires:
  Data Type Conversion/1 -> CAN3_FDC_VCU_VehMalfunLevel_Sta/1
  FDCVCUVehMalfunLevelSta/1 -> Data Type Conversion/1

== system halout/HAL_OUT/CAN3/FD3_VCU0_0x1F0/FDCVMCActStESCYawSta ==
  FDCVMCActStESCYawSta : Inport
  Data Type Conversion : DataTypeConversion  OutDataTypeStr=uint16  RndMeth=Round
  convert_out : FVT_lib/hal/convert_out  gain=0.01  offset=-300
  CAN3_FDC_VMC_ActStESCYaw_Sta : Outport
  wires:
  Data Type Conversion/1 -> CAN3_FDC_VMC_ActStESCYaw_Sta/1
  convert_out/1 -> Data Type Conversion/1
  FDCVMCActStESCYawSta/1 -> convert_out/1

== system halout/HAL_OUT/CAN3/FD3_VCU0_0x1F0/FDCVMCLongAccSta ==
  FDCVMCLongAccSta : Inport
  Data Type Conversion : DataTypeConversion  OutDataTypeStr=uint16  RndMeth=Round
  convert_out : FVT_lib/hal/convert_out  gain=0.001  offset=-20
  CAN3_FDC_VMC_LongAcc_Sta : Outport
  wires:
  Data Type Conversion/1 -> CAN3_FDC_VMC_LongAcc_Sta/1
  convert_out/1 -> Data Type Conversion/1
  FDCVMCLongAccSta/1 -> convert_out/1

== system halout/HAL_OUT/CAN3/FD3_VCU0_0x1F0/FrTqSource ==
  FrTqSource : Inport
  Data Type Conversion : DataTypeConversion  OutDataTypeStr=uint8  RndMeth=Round
  CAN3_Fr_TqSource : Outport
  wires:
  Data Type Conversion/1 -> CAN3_Fr_TqSource/1
  FrTqSource/1 -> Data Type Conversion/1

== system halout/HAL_OUT/CAN3/FD3_VCU0_0x1F0/HVRlyOpFail ==
  HVRlyOpFail : Inport
  Data Type Conversion : DataTypeConversion  OutDataTypeStr=uint8  RndMeth=Round
  CAN3_HVRlyOpFail : Outport
  wires:
  Data Type Conversion/1 -> CAN3_HVRlyOpFail/1
  HVRlyOpFail/1 -> Data Type Conversion/1

== system halout/HAL_OUT/CAN3/FD3_VCU0_0x1F0/HVTHCMSysAvail ==
  HVTHCMSysAvail : Inport
  Data Type Conversion : DataTypeConversion  OutDataTypeStr=uint8  RndMeth=Round
  CAN3_HVTHCMSysAvail : Outport
  wires:
  Data Type Conversion/1 -> CAN3_HVTHCMSysAvail/1
  HVTHCMSysAvail/1 -> Data Type Conversion/1

== system halout/HAL_OUT/CAN3/FD3_VCU0_0x1F0/LVBattChrgtimeAct ==
  LVBattChrgtimeAct : Inport
  Data Type Conversion : DataTypeConversion  OutDataTypeStr=uint16  RndMeth=Round
  CAN3_LVBattChrgtimeAct : Outport
  wires:
  Data Type Conversion/1 -> CAN3_LVBattChrgtimeAct/1
  LVBattChrgtimeAct/1 -> Data Type Conversion/1

== system halout/HAL_OUT/CAN3/FD3_VCU0_0x1F0/LVBattVoltSta ==
  LVBattVoltSta : Inport
  Data Type Conversion : DataTypeConversion  OutDataTypeStr=uint8  RndMeth=Round
  CAN3_LVBattVoltSta : Outport
  wires:
  Data Type Conversion/1 -> CAN3_LVBattVoltSta/1
  LVBattVoltSta/1 -> Data Type Conversion/1

== system halout/HAL_OUT/CAN3/FD3_VCU0_0x1F0/LVChrgHoldTAct ==
  LVChrgHoldTAct : Inport
  Data Type Conversion : DataTypeConversion  OutDataTypeStr=uint16  RndMeth=Round
  CAN3_LVChrgHoldTAct : Outport
  wires:
  Data Type Conversion/1 -> CAN3_LVChrgHoldTAct/1
  LVChrgHoldTAct/1 -> Data Type Conversion/1

== system halout/HAL_OUT/CAN3/FD3_VCU0_0x1F0/LVSilentChrgLv ==
  LVSilentChrgLv : Inport
  Data Type Conversion : DataTypeConversion  OutDataTypeStr=uint8  RndMeth=Round
  CAN3_LVSilentChrgLv : Outport
  wires:
  Data Type Conversion/1 -> CAN3_LVSilentChrgLv/1
  LVSilentChrgLv/1 -> Data Type Conversion/1

== system halout/HAL_OUT/CAN3/FD3_VCU0_0x1F0/LVSilentChrgReq ==
  LVSilentChrgReq : Inport
  Data Type Conversion : DataTypeConversion  OutDataTypeStr=uint8  RndMeth=Round
  CAN3_LVSilentChrgReq : Outport
  wires:
  Data Type Conversion/1 -> CAN3_LVSilentChrgReq/1
  LVSilentChrgReq/1 -> Data Type Conversion/1

== system halout/HAL_OUT/CAN3/FD3_VCU0_0x1F0/LVSilentChrgSta ==
  LVSilentChrgSta : Inport
  Data Type Conversion : DataTypeConversion  OutDataTypeStr=uint8  RndMeth=Round
  CAN3_LVSilentChrgSta : Outport
  wires:
  Data Type Conversion/1 -> CAN3_LVSilentChrgSta/1
  LVSilentChrgSta/1 -> Data Type Conversion/1

== system halout/HAL_OUT/CAN3/FD3_VCU0_0x1F0/MCUActDisFail ==
  MCUActDisFail : Inport
  Data Type Conversion : DataTypeConversion  OutDataTypeStr=uint8  RndMeth=Round
  CAN3_MCUActDisFail : Outport
  wires:
  Data Type Conversion/1 -> CAN3_MCUActDisFail/1
  MCUActDisFail/1 -> Data Type Conversion/1

== system halout/HAL_OUT/CAN3/FD3_VCU0_0x1F0/PMMAllowECUSleep ==
  PMMAllowECUSleep : Inport
  Data Type Conversion : DataTypeConversion  OutDataTypeStr=uint8  RndMeth=Round
  CAN3_PMMAllowECUSleep : Outport
  wires:
  Data Type Conversion/1 -> CAN3_PMMAllowECUSleep/1
  PMMAllowECUSleep/1 -> Data Type Conversion/1

== system halout/HAL_OUT/CAN3/FD3_VCU0_0x1F0/PmicBootReason ==
  PmicBootReason : Inport
  Data Type Conversion : DataTypeConversion  OutDataTypeStr=uint8  RndMeth=Round
  CAN3_PmicBootReason : Outport
  wires:
  Data Type Conversion/1 -> CAN3_PmicBootReason/1
  PmicBootReason/1 -> Data Type Conversion/1

== system halout/HAL_OUT/CAN3/FD3_VCU0_0x1F0/PowerDownFault ==
  PowerDownFault : Inport
  Data Type Conversion : DataTypeConversion  OutDataTypeStr=uint8  RndMeth=Round
  CAN3_PowerDownFault : Outport
  wires:
  Data Type Conversion/1 -> CAN3_PowerDownFault/1
  PowerDownFault/1 -> Data Type Conversion/1

== system halout/HAL_OUT/CAN3/FD3_VCU0_0x1F0/PowerDownState ==
  PowerDownState : Inport
  Data Type Conversion : DataTypeConversion  OutDataTypeStr=uint8  RndMeth=Round
  CAN3_PowerDownState : Outport
  wires:
  Data Type Conversion/1 -> CAN3_PowerDownState/1
  PowerDownState/1 -> Data Type Conversion/1

== system halout/HAL_OUT/CAN3/FD3_VCU0_0x1F0/PowerUpFault ==
  PowerUpFault : Inport
  Data Type Conversion : DataTypeConversion  OutDataTypeStr=uint8  RndMeth=Round
  CAN3_PowerUpFault : Outport
  wires:
  Data Type Conversion/1 -> CAN3_PowerUpFault/1
  PowerUpFault/1 -> Data Type Conversion/1

== system halout/HAL_OUT/CAN3/FD3_VCU0_0x1F0/PowerUpState ==
  PowerUpState : Inport
  Data Type Conversion : DataTypeConversion  OutDataTypeStr=uint8  RndMeth=Round
  CAN3_PowerUpState : Outport
  wires:
  Data Type Conversion/1 -> CAN3_PowerUpState/1
  PowerUpState/1 -> Data Type Conversion/1

== system halout/HAL_OUT/CAN3/FD3_VCU0_0x1F0/PwrDownReq ==
  PwrDownReq : Inport
  Data Type Conversion : DataTypeConversion  OutDataTypeStr=uint8  RndMeth=Round
  CAN3_PwrDownReq : Outport
  wires:
  Data Type Conversion/1 -> CAN3_PwrDownReq/1
  PwrDownReq/1 -> Data Type Conversion/1

== system halout/HAL_OUT/CAN3/FD3_VCU0_0x1F0/PwrStaConstraint ==
  PwrStaConstraint : Inport
  Data Type Conversion : DataTypeConversion  OutDataTypeStr=uint8  RndMeth=Round
  CAN3_PwrStaConstraint : Outport
  wires:
  Data Type Conversion/1 -> CAN3_PwrStaConstraint/1
  PwrStaConstraint/1 -> Data Type Conversion/1

== system halout/HAL_OUT/CAN3/FD3_VCU0_0x1F0/PwrStaONTOIVIPopReq ==
  PwrStaONTOIVIPopReq : Inport
  Data Type Conversion : DataTypeConversion  OutDataTypeStr=uint8  RndMeth=Round
  CAN3_PwrStaONTOIVIPopReq : Outport
  wires:
  Data Type Conversion/1 -> CAN3_PwrStaONTOIVIPopReq/1
  PwrStaONTOIVIPopReq/1 -> Data Type Conversion/1

== system halout/HAL_OUT/CAN3/FD3_VCU0_0x1F0/PwrStaONTOIVIPopT ==
  PwrStaONTOIVIPopT : Inport
  Data Type Conversion : DataTypeConversion  OutDataTypeStr=uint16  RndMeth=Round
  CAN3_PwrStaONTOIVIPopT : Outport
  wires:
  Data Type Conversion/1 -> CAN3_PwrStaONTOIVIPopT/1
  PwrStaONTOIVIPopT/1 -> Data Type Conversion/1

== system halout/HAL_OUT/CAN3/FD3_VCU0_0x1F0/PwrStaSelect ==
  PwrStaSelect : Inport
  Data Type Conversion : DataTypeConversion  OutDataTypeStr=uint8  RndMeth=Round
  CAN3_PwrStaSelect : Outport
  wires:
  Data Type Conversion/1 -> CAN3_PwrStaSelect/1
  PwrStaSelect/1 -> Data Type Conversion/1

== system halout/HAL_OUT/CAN3/FD3_VCU0_0x1F0/PwrStaTOSta ==
  PwrStaTOSta : Inport
  Data Type Conversion : DataTypeConversion  OutDataTypeStr=uint8  RndMeth=Round
  CAN3_PwrStaTOSta : Outport
  wires:
  Data Type Conversion/1 -> CAN3_PwrStaTOSta/1
  PwrStaTOSta/1 -> Data Type Conversion/1

== system halout/HAL_OUT/CAN3/FD3_VCU0_0x1F0/PwrUpReq ==
  PwrUpReq : Inport
  Data Type Conversion : DataTypeConversion  OutDataTypeStr=uint8  RndMeth=Round
  CAN3_PwrUpReq : Outport
  wires:
  Data Type Conversion/1 -> CAN3_PwrUpReq/1
  PwrUpReq/1 -> Data Type Conversion/1

== system halout/HAL_OUT/CAN3/FD3_VCU0_0x1F0/RrTqSource ==
  RrTqSource : Inport
  Data Type Conversion : DataTypeConversion  OutDataTypeStr=uint8  RndMeth=Round
  CAN3_Rr_TqSource : Outport
  wires:
  Data Type Conversion/1 -> CAN3_Rr_TqSource/1
  RrTqSource/1 -> Data Type Conversion/1

== system halout/HAL_OUT/CAN3/FD3_VCU0_0x1F0/SchedChgTOSta ==
  SchedChgTOSta : Inport
  Data Type Conversion : DataTypeConversion  OutDataTypeStr=uint8  RndMeth=Round
  CAN3_SchedChgTOSta : Outport
  wires:
  Data Type Conversion/1 -> CAN3_SchedChgTOSta/1
  SchedChgTOSta/1 -> Data Type Conversion/1

== system halout/HAL_OUT/CAN3/FD3_VCU0_0x1F0/SilentChkAllowSleep ==
  SilentChkAllowSleep : Inport
  Data Type Conversion : DataTypeConversion  OutDataTypeStr=uint8  RndMeth=Round
  CAN3_SilentChkAllowSleep : Outport
  wires:
  Data Type Conversion/1 -> CAN3_SilentChkAllowSleep/1
  SilentChkAllowSleep/1 -> Data Type Conversion/1

== system halout/HAL_OUT/CAN3/FD3_VCU0_0x1F0/Subsystem ==
  s8_AcoreReadyToSleep : Inport
  VOUTP_CurrentNmState_enum : Inport  Port=2
  VOUTP_OTAPwrReqOFFChkSta_enum : Inport  Port=3
  VOUTP_OTAPwrReqStdChkSta_enum : Inport  Port=4
  Bitwise AND : simulink/Logic and Bit Operations/Bitwise Operator  logicop=AND  UseBitMask=on  BitMask=bin2dec('11111111')  BitMaskRealWorld=Stored Integer
  Bitwise AND1 : simulink/Logic and Bit Operations/Bitwise Operator  logicop=AND  UseBitMask=on  BitMask=bin2dec('11111111')  BitMaskRealWorld=Stored Integer
  Bitwise AND2 : simulink/Logic and Bit Operations/Bitwise Operator  logicop=AND  UseBitMask=on  BitMask=bin2dec('11111111')  BitMaskRealWorld=Stored Integer
  Bitwise OR2 : simulink/Logic and Bit Operations/Bitwise Operator  logicop=OR  UseBitMask=off  NumInputPorts=4  BitMask=bin2dec('00000000000000000000')  BitMaskRealWorld=Stored Integer
  Gain : Gain  Gain=50  OutDataTypeStr=single
  Saturation : Saturate  UpperLimit=1  LowerLimit=0  OutDataTypeStr=uint8
  Saturation1 : Saturate  UpperLimit=7  LowerLimit=0  OutDataTypeStr=uint8
  Saturation2 : Saturate  UpperLimit=3  LowerLimit=0  OutDataTypeStr=uint8
  Saturation3 : Saturate  UpperLimit=3  LowerLimit=0  OutDataTypeStr=uint8
  Shift Arithmetic6 : ArithShift  BitShiftNumber=1  BitShiftDirection=Left
  Shift Arithmetic7 : ArithShift  BitShiftNumber=4  BitShiftDirection=Left
  Shift Arithmetic8 : ArithShift  BitShiftNumber=6  BitShiftDirection=Left
  VehHVPwrAvail4THCM : Outport
  wires:
  s8_AcoreReadyToSleep/1 -> Saturation/1
  VOUTP_CurrentNmState_enum/1 -> Saturation1/1
  VOUTP_OTAPwrReqOFFChkSta_enum/1 -> Saturation2/1
  VOUTP_OTAPwrReqStdChkSta_enum/1 -> Saturation3/1
  Bitwise OR2/1 -> Gain/1
  Gain/1 -> VehHVPwrAvail4THCM/1
  Saturation1/1 -> Shift Arithmetic6/1
  Saturation/1 -> Bitwise OR2/1
  Saturation2/1 -> Shift Arithmetic7/1
  Saturation3/1 -> Shift Arithmetic8/1
  Shift Arithmetic8/1 -> Bitwise AND/1
  Bitwise AND/1 -> Bitwise OR2/4
  Shift Arithmetic7/1 -> Bitwise AND1/1
  Bitwise AND1/1 -> Bitwise OR2/3
  Shift Arithmetic6/1 -> Bitwise AND2/1
  Bitwise AND2/1 -> Bitwise OR2/2

== system halout/HAL_OUT/CAN3/FD3_VCU0_0x1F0/SysAllowReadySta ==
  SysAllowReadySta : Inport
  Data Type Conversion : DataTypeConversion  OutDataTypeStr=uint8  RndMeth=Round
  CAN3_SysAllowReadySta : Outport
  wires:
  Data Type Conversion/1 -> CAN3_SysAllowReadySta/1
  SysAllowReadySta/1 -> Data Type Conversion/1

== system halout/HAL_OUT/CAN3/FD3_VCU0_0x1F0/SysPwrSta ==
  SysPwrSta : Inport
  Data Type Conversion : DataTypeConversion  OutDataTypeStr=uint8  RndMeth=Round
  CAN3_SysPwrSta : Outport
  wires:
  Data Type Conversion/1 -> CAN3_SysPwrSta/1
  SysPwrSta/1 -> Data Type Conversion/1

== system halout/HAL_OUT/CAN3/FD3_VCU0_0x1F0/TCountSta ==
  TCountSta : Inport
  Data Type Conversion : DataTypeConversion  OutDataTypeStr=uint8  RndMeth=Round
  CAN3_TCountSta : Outport
  wires:
  Data Type Conversion/1 -> CAN3_TCountSta/1
  TCountSta/1 -> Data Type Conversion/1

== system halout/HAL_OUT/CAN3/FD3_VCU0_0x1F0/TimerAllowSleep ==
  TimerAllowSleep : Inport
  Data Type Conversion : DataTypeConversion  OutDataTypeStr=uint8  RndMeth=Round
  CAN3_TimerAllowSleep : Outport
  wires:
  Data Type Conversion/1 -> CAN3_TimerAllowSleep/1
  TimerAllowSleep/1 -> Data Type Conversion/1

== system halout/HAL_OUT/CAN3/FD3_VCU0_0x1F0/VCUBrkSWSta ==
  VCUBrkSWSta : Inport
  Data Type Conversion : DataTypeConversion  OutDataTypeStr=uint8  RndMeth=Round
  CAN3_VCUBrkSWSta : Outport
  wires:
  Data Type Conversion/1 -> CAN3_VCUBrkSWSta/1
  VCUBrkSWSta/1 -> Data Type Conversion/1

== system halout/HAL_OUT/CAN3/FD3_VCU0_0x1F0/VCUFLDoorSta ==
  VCUFLDoorSta : Inport
  Data Type Conversion : DataTypeConversion  OutDataTypeStr=uint8  RndMeth=Round
  CAN3_VCUFLDoorSta : Outport
  wires:
  Data Type Conversion/1 -> CAN3_VCUFLDoorSta/1
  VCUFLDoorSta/1 -> Data Type Conversion/1

== system halout/HAL_OUT/CAN3/FD3_VCU0_0x1F0/VCUFRDoorSta ==
  VCUFRDoorSta : Inport
  Data Type Conversion : DataTypeConversion  OutDataTypeStr=uint8  RndMeth=Round
  CAN3_VCUFRDoorSta : Outport
  wires:
  Data Type Conversion/1 -> CAN3_VCUFRDoorSta/1
  VCUFRDoorSta/1 -> Data Type Conversion/1

== system halout/HAL_OUT/CAN3/FD3_VCU0_0x1F0/VCURLDoorSta ==
  VCURLDoorSta : Inport
  Data Type Conversion : DataTypeConversion  OutDataTypeStr=uint8  RndMeth=Round
  CAN3_VCURLDoorSta : Outport
  wires:
  Data Type Conversion/1 -> CAN3_VCURLDoorSta/1
  VCURLDoorSta/1 -> Data Type Conversion/1

== system halout/HAL_OUT/CAN3/FD3_VCU0_0x1F0/VCURRDoorSta ==
  VCURRDoorSta : Inport
  Data Type Conversion : DataTypeConversion  OutDataTypeStr=uint8  RndMeth=Round
  CAN3_VCURRDoorSta : Outport
  wires:
  Data Type Conversion/1 -> CAN3_VCURRDoorSta/1
  VCURRDoorSta/1 -> Data Type Conversion/1

== system halout/HAL_OUT/CAN3/FD3_VCU0_0x1F0/VehHVPwrAvail4THCM ==
  VehHVPwrAvail4THCM : Inport
  Data Type Conversion : DataTypeConversion  OutDataTypeStr=uint8  RndMeth=Round
  convert_out : FVT_lib/hal/convert_out  gain=50  offset=0
  CAN3_VehHVPwrAvail4THCM : Outport
  wires:
  Data Type Conversion/1 -> CAN3_VehHVPwrAvail4THCM/1
  convert_out/1 -> Data Type Conversion/1
  VehHVPwrAvail4THCM/1 -> convert_out/1

== system halout/HAL_OUT/CAN3/FD3_VCU0_0x1F0/WisrBootReason ==
  WisrBootReason : Inport
  Data Type Conversion : DataTypeConversion  OutDataTypeStr=uint32  RndMeth=Round
  CAN3_WisrBootReason : Outport
  wires:
  Data Type Conversion/1 -> CAN3_WisrBootReason/1
  WisrBootReason/1 -> Data Type Conversion/1

== system halout/HAL_OUT/CAN3/FD3_VCU1_0x115/APSStaSystem ==
  APSStaSystem : Inport
  Data Type Conversion : DataTypeConversion  OutDataTypeStr=uint8  RndMeth=Round
  CAN3_APS_Sta_System : Outport
  wires:
  Data Type Conversion/1 -> CAN3_APS_Sta_System/1
  APSStaSystem/1 -> Data Type Conversion/1

== system halout/HAL_OUT/CAN3/FD3_VCU1_0x115/ActiveDischReq ==
  ActiveDischReq : Inport
  Data Type Conversion : DataTypeConversion  OutDataTypeStr=uint8  RndMeth=Round
  CAN3_ActiveDischReq : Outport
  wires:
  Data Type Conversion/1 -> CAN3_ActiveDischReq/1
  ActiveDischReq/1 -> Data Type Conversion/1

== system halout/HAL_OUT/CAN3/FD3_VCU1_0x115/CSVCU1 ==
  CSVCU1 : Inport
  Data Type Conversion : DataTypeConversion  OutDataTypeStr=uint8  RndMeth=Round
  CAN3_CS_VCU1 : Outport
  wires:
  Data Type Conversion/1 -> CAN3_CS_VCU1/1
  CSVCU1/1 -> Data Type Conversion/1

== system halout/HAL_OUT/CAN3/FD3_VCU1_0x115/CoastDwModeStaChk ==
  CoastDwModeStaChk : Inport
  Data Type Conversion : DataTypeConversion  OutDataTypeStr=uint8  RndMeth=Round
  CAN3_CoastDwModeStaChk : Outport
  wires:
  Data Type Conversion/1 -> CAN3_CoastDwModeStaChk/1
  CoastDwModeStaChk/1 -> Data Type Conversion/1

== system halout/HAL_OUT/CAN3/FD3_VCU1_0x115/DCDCEnaReq ==
  DCDCEnaReq : Inport
  Data Type Conversion : DataTypeConversion  OutDataTypeStr=uint8  RndMeth=Round
  CAN3_DCDCEnaReq : Outport
  wires:
  Data Type Conversion/1 -> CAN3_DCDCEnaReq/1
  DCDCEnaReq/1 -> Data Type Conversion/1

== system halout/HAL_OUT/CAN3/FD3_VCU1_0x115/DCDCVoltSetpoint ==
  DCDCVoltSetpoint : Inport
  Data Type Conversion : DataTypeConversion  OutDataTypeStr=uint8  RndMeth=Round
  convert_out : FVT_lib/hal/convert_out  gain=0.0235  offset=12
  CAN3_DCDCVoltSetpoint : Outport
  wires:
  Data Type Conversion/1 -> CAN3_DCDCVoltSetpoint/1
  convert_out/1 -> Data Type Conversion/1
  DCDCVoltSetpoint/1 -> convert_out/1

== system halout/HAL_OUT/CAN3/FD3_VCU1_0x115/DemoModeStaChk ==
  DemoModeStaChk : Inport
  Data Type Conversion : DataTypeConversion  OutDataTypeStr=uint8  RndMeth=Round
  CAN3_DemoModeStaChk : Outport
  wires:
  Data Type Conversion/1 -> CAN3_DemoModeStaChk/1
  DemoModeStaChk/1 -> Data Type Conversion/1

== system halout/HAL_OUT/CAN3/FD3_VCU1_0x115/DrSeatSta ==
  DrSeatSta : Inport
  Data Type Conversion : DataTypeConversion  OutDataTypeStr=uint8  RndMeth=Round
  CAN3_Dr_SeatSta : Outport
  wires:
  Data Type Conversion/1 -> CAN3_Dr_SeatSta/1
  DrSeatSta/1 -> Data Type Conversion/1

== system halout/HAL_OUT/CAN3/FD3_VCU1_0x115/DynoModeStaChk ==
  DynoModeStaChk : Inport
  Data Type Conversion : DataTypeConversion  OutDataTypeStr=uint8  RndMeth=Round
  CAN3_DynoModeStaChk : Outport
  wires:
  Data Type Conversion/1 -> CAN3_DynoModeStaChk/1
  DynoModeStaChk/1 -> Data Type Conversion/1

== system halout/HAL_OUT/CAN3/FD3_VCU1_0x115/HVBatCnctReq ==
  HVBatCnctReq : Inport
  Data Type Conversion : DataTypeConversion  OutDataTypeStr=uint8  RndMeth=Round
  CAN3_HVBatCnctReq : Outport
  wires:
  Data Type Conversion/1 -> CAN3_HVBatCnctReq/1
  HVBatCnctReq/1 -> Data Type Conversion/1

== system halout/HAL_OUT/CAN3/FD3_VCU1_0x115/HVSysReadyToCharge ==
  HVSysReadyToCharge : Inport
  Data Type Conversion : DataTypeConversion  OutDataTypeStr=uint8  RndMeth=Round
  CAN3_HVSysReadyToCharge : Outport
  wires:
  Data Type Conversion/1 -> CAN3_HVSysReadyToCharge/1
  HVSysReadyToCharge/1 -> Data Type Conversion/1

== system halout/HAL_OUT/CAN3/FD3_VCU1_0x115/LVChrgFuncStaChk ==
  LVChrgFuncStaChk : Inport
  Data Type Conversion : DataTypeConversion  OutDataTypeStr=uint8  RndMeth=Round
  CAN3_LVChrgFuncStaChk : Outport
  wires:
  Data Type Conversion/1 -> CAN3_LVChrgFuncStaChk/1
  LVChrgFuncStaChk/1 -> Data Type Conversion/1

== system halout/HAL_OUT/CAN3/FD3_VCU1_0x115/MSACrlSta ==
  MSACrlSta : Inport
  Data Type Conversion : DataTypeConversion  OutDataTypeStr=uint8  RndMeth=Round
  CAN3_MSA_Crl_Sta : Outport
  wires:
  Data Type Conversion/1 -> CAN3_MSA_Crl_Sta/1
  MSACrlSta/1 -> Data Type Conversion/1

== system halout/HAL_OUT/CAN3/FD3_VCU1_0x115/PButtonSta ==
  PButtonSta : Inport
  Data Type Conversion : DataTypeConversion  OutDataTypeStr=uint8  RndMeth=Round
  CAN3_P_Button_Sta : Outport
  wires:
  Data Type Conversion/1 -> CAN3_P_Button_Sta/1
  PButtonSta/1 -> Data Type Conversion/1

== system halout/HAL_OUT/CAN3/FD3_VCU1_0x115/PrkReq ==
  PrkReq : Inport
  Data Type Conversion : DataTypeConversion  OutDataTypeStr=uint8  RndMeth=Round
  CAN3_PrkReq : Outport
  wires:
  Data Type Conversion/1 -> CAN3_PrkReq/1
  PrkReq/1 -> Data Type Conversion/1

== system halout/HAL_OUT/CAN3/FD3_VCU1_0x115/PrkReqValid ==
  PrkReqValid : Inport
  Data Type Conversion : DataTypeConversion  OutDataTypeStr=uint8  RndMeth=Round
  CAN3_PrkReqValid : Outport
  wires:
  Data Type Conversion/1 -> CAN3_PrkReqValid/1
  PrkReqValid/1 -> Data Type Conversion/1

== system halout/HAL_OUT/CAN3/FD3_VCU1_0x115/PwrSta ==
  PwrSta : Inport
  Data Type Conversion : DataTypeConversion  OutDataTypeStr=uint8  RndMeth=Round
  CAN3_PwrSta : Outport
  wires:
  Data Type Conversion/1 -> CAN3_PwrSta/1
  PwrSta/1 -> Data Type Conversion/1

== system halout/HAL_OUT/CAN3/FD3_VCU1_0x115/RCVCU1 ==
  RCVCU1 : Inport
  Data Type Conversion : DataTypeConversion  OutDataTypeStr=uint8  RndMeth=Round
  CAN3_RC_VCU1 : Outport
  wires:
  Data Type Conversion/1 -> CAN3_RC_VCU1/1
  RCVCU1/1 -> Data Type Conversion/1

== system halout/HAL_OUT/CAN3/FD3_VCU1_0x115/ShiftGearPosn ==
  ShiftGearPosn : Inport
  Data Type Conversion : DataTypeConversion  OutDataTypeStr=uint8  RndMeth=Round
  CAN3_ShiftGearPosn : Outport
  wires:
  Data Type Conversion/1 -> CAN3_ShiftGearPosn/1
  ShiftGearPosn/1 -> Data Type Conversion/1

== system halout/HAL_OUT/CAN3/FD3_VCU1_toNIDEC_0x116/ActiveDischReqtoNidec ==
  ActiveDischReqtoNidec : Inport
  Data Type Conversion : DataTypeConversion  OutDataTypeStr=uint8  RndMeth=Round
  CAN3_ActiveDischReq_toNidec : Outport
  wires:
  Data Type Conversion/1 -> CAN3_ActiveDischReq_toNidec/1
  ActiveDischReqtoNidec/1 -> Data Type Conversion/1

== system halout/HAL_OUT/CAN3/FD3_VCU1_toNIDEC_0x116/CSVCU1toNidec ==
  CSVCU1toNidec : Inport
  Data Type Conversion : DataTypeConversion  OutDataTypeStr=uint8  RndMeth=Round
  CAN3_CS_VCU1_toNidec : Outport
  wires:
  Data Type Conversion/1 -> CAN3_CS_VCU1_toNidec/1
  CSVCU1toNidec/1 -> Data Type Conversion/1

== system halout/HAL_OUT/CAN3/FD3_VCU1_toNIDEC_0x116/CoastDwModeStaChktoNidec ==
  CoastDwModeStaChktoNidec : Inport
  Data Type Conversion : DataTypeConversion  OutDataTypeStr=uint8  RndMeth=Round
  CAN3_CoastDwModeStaChk_toNidec : Outport
  wires:
  Data Type Conversion/1 -> CAN3_CoastDwModeStaChk_toNidec/1
  CoastDwModeStaChktoNidec/1 -> Data Type Conversion/1
